simulink model "get_phi"  (R2013a)
settings: Solver=ode45  StartTime=0.0  StopTime=10.0  RelTol=1e-3
libraries: cstblocks x2
settings Model: Creator=Christoph Zech  LastModifiedBy=Christoph Zech

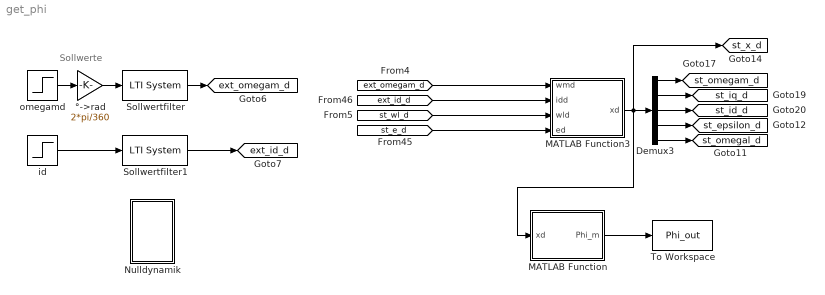
== system get_phi ==
  note: Sollwerte
  Demux3 : Demux  Outputs=5
  MATLAB Function : MATLAB Function  TreatAsAtomicUnit=on
  MATLAB Function3 : MATLAB Function  TreatAsAtomicUnit=on
  Nulldynamik : Subsystem
  Sollwertfilter : cstblocks/LTI System  sys=parReg.ssSF  IC=[]
  Sollwertfilter1 : cstblocks/LTI System  sys=parReg.ssSFi  IC=[]
  To Workspace : ToWorkspace  VariableName=Phi_out  SampleTime=-1  SaveFormat=Timeseries
  id : Step  Time=0.5  After=0.1  SampleTime=0
  omegamd : Step  Time=2  After=1000/60*360  SampleTime=0
  °->rad : Gain  Gain=2*pi/360
  tag scope: ext_id_d=global, ext_omegam_d=global, st_epsilon_d=global, st_id_d=global, st_iq_d=global, st_omegal_d=global, st_omegam_d=global, st_x_d=global
  wires:
  °->rad/1 -> Sollwertfilter/1
  Sollwertfilter/1 -> [ext_omegam_d]
  Sollwertfilter1/1 -> [ext_id_d]
  id/1 -> Sollwertfilter1/1
  omegamd/1 -> °->rad/1
  MATLAB Function3/1(xd) -> MATLAB Function/1(xd), [st_x_d], Demux3/1
  Demux3/4 -> [st_epsilon_d]
  Demux3/5 -> [st_omegal_d]
  Demux3/1 -> [st_omegam_d]
  Demux3/2 -> [st_iq_d]
  Demux3/3 -> [st_id_d]
  [ext_omegam_d] -> MATLAB Function3/1(wmd)
  [st_wl_d] -> MATLAB Function3/3(wld)
  [st_e_d] -> MATLAB Function3/4(ed)
  [ext_id_d] -> MATLAB Function3/2(idd)
  MATLAB Function/1(Phi_m) -> To Workspace/1

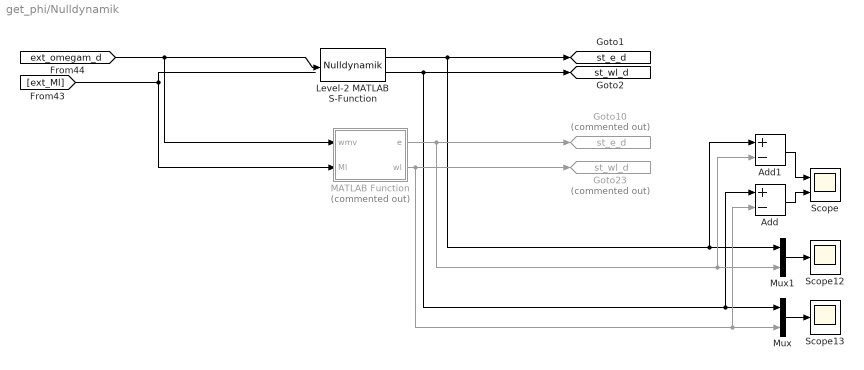
== system get_phi/Nulldynamik ==
  Add : Sum  Inputs=+-
  Add1 : Sum  Inputs=+-
  Goto10 : Goto  Commented=on  GotoTag=st_e_d  TagVisibility=global
  Goto23 : Goto  Commented=on  GotoTag=st_wl_d  TagVisibility=global
  Level-2 MATLAB S-Function : M-S-Function  FunctionName=Nulldynamik  Parameters=parSys.epsilon_0 parSys.omegal_0 [parSys.cr1 parSys.cr3 parSys.rl parSys.rm parSys.dl parSys.Il]
  MATLAB Function : MATLAB Function  Commented=on  TreatAsAtomicUnit=on
  Mux : Mux  Inputs=2
  Mux1 : Mux  Inputs=2
  Scope : Scope  NumInputPorts=2
      settings: YMin=-4.5e-05~-0.275  YMax=5e-05~0.075  SaveName=ScopeData14
  Scope12 : Scope
      settings: YMin=-0.014  YMax=0.008  SaveName=ScopeData12
  Scope13 : Scope
      settings: SaveName=ScopeData13
  tag scope: st_e_d=global, st_wl_d=global
  wires:
  [ext_Ml] -> MATLAB Function/2(Ml)
  Level-2 MATLAB S-Function/1 -> Add1/1, Mux1/1, [st_e_d]
  Level-2 MATLAB S-Function/2 -> Add/1, Mux/1, [st_wl_d]
  [ext_omegam_d] -> MATLAB Function/1(wmv), Level-2 MATLAB S-Function/1
  MATLAB Function/1(e) -> Add1/2, Mux1/2, Goto10/1
  MATLAB Function/2(wl) -> Add/2, Mux/2, Goto23/1
  Mux/1 -> Scope13/1
  Mux1/1 -> Scope12/1
  Add/1 -> Scope/2
  Add1/1 -> Scope/1

== matlab function get_phi/MATLAB Function ==
  settings: updateMethod=DISCRETE  sampleTime=parSys.TsID
  data: xd input; Phi_m output
function Phi_m = fcn(xd)
%#codegen
%Parameter
I_l  = 4e-5;     %Trägheitsmoment Last
cr1 = 10;       %lineare Steifigkeit Riemen
cr3 = 1e6;      %kubische Steifigkeit Riemen (1e6)
dl  = 0.001;    %visk. Dämpfung Last
rl  = 0.05;     %Radius Riemenscheibe Last
I_m  = 0.5e-5;   %Trägheitsmoment Motor
dm  = 0.01;     %viskose Dämpfung Motor
rm  = 0.025;    %Radius Riemenscheibe Motor
Rm  = 1.388;    %Widerstand PSM
Lm  = 1.475e-3; %Induktivität PSM
p   = 2.0;      %Polpaarzahl PSM
Phi = 2.715e-2; %Fluss Permanentmagnet PSM

Ta = 0.1e-3;

wm_d = xd(1);
iq_d = xd(2);
id_d = xd(3);
e_d = xd(4);
wl_d = xd(5);

Phi_m = [1 - Ta * dm / I_m 0.3e1 / 0.2e1 * Ta * Phi * p / I_m 0 (Ta * (12 * cr3 * e_d ^ 2 * rm + 4 * cr1 * rm) / I_m) / 0.2e1 0 0 0; (Ta * (3 * Lm * id_d * p - 2 * Phi * p) / Lm) / 0.3e1 0.1e1 - 0.2e1 / 0.3e1 * Ta * Rm / Lm Ta * p * wm_d 0 0 0 0; -Ta * iq_d * p -Ta * p * wm_d 0.1e1 - 0.2e1 / 0.3e1 * Ta * Rm / Lm 0 0 0 0; -Ta * rm 0 0 1 Ta * rl 0 0; 0 0 0 -Ta * (6 * cr3 * e_d ^ 2 * rl + 2 * cr1 * rl) / I_l 1 - Ta * dl / I_l 0 0; Ta 0 0 0 0 1 0; 0 0 Ta 0 0 0 1;];
end

== matlab function get_phi/Nulldynamik/MATLAB Function ==
  settings: updateMethod=DISCRETE  sampleTime=parSys.TsID
  data: wmv input; e output; Ml input; wl output; parSys parameter
function [e, wl] = Nulldynamik_diskret(wmv, Ml, parSys)
%#codegen
persistent k
persistent x1
persistent x2

wm = wmv(1);

if (isempty(k))
    k = 0;
end
if (isempty(x1))
    x1 = parSys.epsilon_0;
end
if (isempty(x2))
    x2 = parSys.omegal_0;
end

cr1 = parSys.cr1;
cr3 = parSys.cr3;
Il = parSys.Il;
rl = parSys.rl;
rm = parSys.rm;
dl = parSys.dl;

k = k + parSys.TsID;

f1 = rl*x2-rm*wm;
f2 = 1/Il*(-2*(cr1*x1+cr3*x1^3)*rl - dl*x2 + Ml);

xp1 = x1 + parSys.TsID*f1;
xp2 = x2 + parSys.TsID*f2;

x1 = x1 + parSys.TsID/2*(f1 + (rl*xp2 - rm*wm));
x2  = x2 + parSys.TsID/2*(f2 + 1/Il*(-2*(cr1*xp1 + cr3*xp1^3)*rl - dl*xp2 + Ml));

e = x1;
wl = x2;
end

== matlab function get_phi/MATLAB Function3 ==
  settings: updateMethod=DISCRETE  sampleTime=parSys.TsID
  data: wmd input; idd input; xd output; wld input; ed input; parSys parameter
function xd  = fcn(wmd, idd, wld, ed, parSys)
%#codegen
wm = wmd(1);
wmp = wmd(2);
wmpp = wmd(3);
id = idd(1);
idp = idd(2);
wl = wld;
e = ed;

%parameter;
%Zuweisungen
Lm = parSys.Lm;
Rm = parSys.Rm;
cr1 = parSys.cr1;
cr3 = parSys.cr3;
rm = parSys.rm;
dm = parSys.dm;
rl = parSys.rl;
dl = parSys.dl;
I_l = parSys.Il;
I_m = parSys.Im;
p = parSys.p;
Phi = parSys.Phi;

iq = 0.2e1 / 0.3e1 * (-2 * cr3 * e ^ 3 * rm - 2 * cr1 * e * rm + wmp * I_m + dm * wm) / Phi / p;

xd = [wm iq id e wl];


end
